simulink model "bhaaa"  (R2016b)
settings: Solver=ode15s  StartTime=0.0  StopTime=30  FixedStep=0.001  RelTol=1e-5  EnableMultiTasking=on
undefined symbols (not defined in the file): b1_damp, b2_damp, b3_damp, b4_damp, g, Hz, L1x, L1y, L1z, L2x, L2y, L2z, L3x, L3y, L3z, mass1, mass2, mass3, mass4, Rturn, sigbuilder_block, theta1_0, theta1_dot_0, theta2_0, theta2_dot_0, theta3_0, theta3_dot_0, theta4_0, theta4_dot_0, X, Y, Z
libraries: sm_lib x26, nesl_utility x17
(part 2 of 2)

== matlab function bhaaa/SIMULINK_MODEL/inside_MCKGQ/MCKGQ ==
  data: L1X_s input; M output; L2X_s input; L3X_s input; L1Y_s input; L2Y_s input; L3Y_s input; L1Z_s input; L2Z_s input; L3Z_s input; R4_s input; TH1_s input; TH2_s input; TH3_s input; TH1_s_D input; TH2_s_D input; TH3_s_D input; TH4_s_D input; b1_s input; b2_s input; b3_s input; b4_s input; g_s input; m1_s input; m2_s input; m3_s input; m4_s input; taum1_s input; taum2_s input; taum3_s input; taum4_s input; C output; K output; G output; Q output
function [M,C,K,G,Q] = MCKGQ(L1X_s,L2X_s,L3X_s,L1Y_s,L2Y_s,L3Y_s,L1Z_s,L2Z_s,L3Z_s,R4_s,TH1_s,TH2_s,TH3_s,TH1_s_D,TH2_s_D,TH3_s_D,TH4_s_D,b1_s,b2_s,b3_s,b4_s,g_s,m1_s,m2_s,m3_s,m4_s,taum1_s,taum2_s,taum3_s,taum4_s)
%#codegen

%    This function was generated by the Symbolic Math Toolbox version 7.0.
%    13-Sep-2016 13:01:16

M = reshape([L1Y_s.^2.*m1_s.*(1.0./3.0)+L1Y_s.^2.*m2_s+L1Y_s.^2.*m3_s+L2Y_s.^2.*m2_s.*(1.0./3.0)+L2Y_s.^2.*m3_s+L3Y_s.^2.*m3_s.*(1.0./3.0)+L1Z_s.^2.*m1_s.*(1.0./1.2e1)+L2Z_s.^2.*m2_s.*(1.0./1.2e1)+L3Z_s.^2.*m3_s.*(1.0./1.2e1)+L1Y_s.*L2Y_s.*m2_s.*cos(TH2_s)+L1Y_s.*L2Y_s.*m3_s.*cos(TH2_s).*2.0+L2Y_s.*L3Y_s.*m3_s.*cos(TH3_s)+L1Y_s.*L3Y_s.*m3_s.*cos(TH2_s+TH3_s),L2Y_s.^2.*m2_s.*(1.0./3.0)+L2Y_s.^2.*m3_s+L3Y_s.^2.*m3_s.*(1.0./3.0)+L2Z_s.^2.*m2_s.*(1.0./1.2e1)+L3Z_s.^2.*m3_s.*(1.0./1.2e1)+L1Y_s.*L2Y_s.*m2_s.*cos(TH2_s).*(1.0./2.0)+L1Y_s.*L2Y_s.*m3_s.*cos(TH2_s)+L2Y_s.*L3Y_s.*m3_s.*cos(TH3_s)+L1Y_s.*L3Y_s.*m3_s.*cos(TH2_s+TH3_s).*(1.0./2.0),m3_s.*(L3Y_s.^2.*4.0+L3Z_s.^2+L1Y_s.*L3Y_s.*cos(TH2_s+TH3_s).*6.0+L2Y_s.*L3Y_s.*cos(TH3_s).*6.0).*(1.0./1.2e1),0.0,L2Y_s.^2.*m2_s.*(1.0./3.0)+L2Y_s.^2.*m3_s+L3Y_s.^2.*m3_s.*(1.0./3.0)+L2Z_s.^2.*m2_s.*(1.0./1.2e1)+L3Z_s.^2.*m3_s.*(1.0./1.2e1)+L1Y_s.*L2Y_s.*m2_s.*cos(TH2_s).*(1.0./2.0)+L1Y_s.*L2Y_s.*m3_s.*cos(TH2_s)+L2Y_s.*L3Y_s.*m3_s.*cos(TH3_s)+L1Y_s.*L3Y_s.*m3_s.*cos(TH2_s+TH3_s).*(1.0./2.0),L2Y_s.^2.*m2_s.*(1.0./3.0)+L2Y_s.^2.*m3_s+L3Y_s.^2.*m3_s.*(1.0./3.0)+L2Z_s.^2.*m2_s.*(1.0./1.2e1)+L3Z_s.^2.*m3_s.*(1.0./1.2e1)+L2Y_s.*L3Y_s.*m3_s.*cos(TH3_s),m3_s.*(L3Y_s.^2.*4.0+L3Z_s.^2+L2Y_s.*L3Y_s.*cos(TH3_s).*6.0).*(1.0./1.2e1),0.0,m3_s.*(L3Y_s.^2.*4.0+L3Z_s.^2+L1Y_s.*L3Y_s.*cos(TH2_s+TH3_s).*6.0+L2Y_s.*L3Y_s.*cos(TH3_s).*6.0).*(1.0./1.2e1),m3_s.*(L3Y_s.^2.*4.0+L3Z_s.^2+L2Y_s.*L3Y_s.*cos(TH3_s).*6.0).*(1.0./1.2e1),m3_s.*(L3Y_s.^2.*4.0+L3Z_s.^2).*(1.0./1.2e1),0.0,0.0,0.0,0.0,L1X_s.^2.*m1_s.*(1.0./1.2e1)+L2X_s.^2.*m2_s.*(1.0./1.2e1)+L3X_s.^2.*m3_s.*(1.0./1.2e1)+L1Y_s.^2.*m1_s.*(1.0./6.0)+L1Y_s.^2.*m2_s.*(1.0./2.0)+L1Y_s.^2.*m3_s.*(1.0./2.0)+L2Y_s.^2.*m2_s.*(1.0./6.0)+L2Y_s.^2.*m3_s.*(1.0./2.0)+L3Y_s.^2.*m3_s.*(1.0./6.0)+L1Z_s.^2.*m1_s.*(1.0./2.4e1)+L2Z_s.^2.*m2_s.*(1.0./2.4e1)+L3Z_s.^2.*m3_s.*(1.0./2.4e1)+R4_s.^2.*m4_s.*(1.0./2.0)+L3Y_s.^2.*m3_s.*cos(TH1_s.*2.0+TH2_s.*2.0+TH3_s.*2.0).*(1.0./6.0)-L3Z_s.^2.*m3_s.*cos(TH1_s.*2.0+TH2_s.*2.0+TH3_s.*2.0).*(1.0./2.4e1)+L1Y_s.^2.*m1_s.*cos(TH1_s.*2.0).*(1.0./6.0)+L1Y_s.^2.*m2_s.*cos(TH1_s.*2.0).*(1.0./2.0)+L1Y_s.^2.*m3_s.*cos(TH1_s.*2.0).*(1.0./2.0)-L1Z_s.^2.*m1_s.*cos(TH1_s.*2.0).*(1.0./2.4e1)+L2Y_s.^2.*m2_s.*cos(TH1_s.*2.0+TH2_s.*2.0).*(1.0./6.0)+L2Y_s.^2.*m3_s.*cos(TH1_s.*2.0+TH2_s.*2.0).*(1.0./2.0)-L2Z_s.^2.*m2_s.*cos(TH1_s.*2.0+TH2_s.*2.0).*(1.0./2.4e1)+L1Y_s.*L2Y_s.*m2_s.*cos(TH2_s).*(1.0./2.0)+L1Y_s.*L2Y_s.*m3_s.*cos(TH2_s)+L2Y_s.*L3Y_s.*m3_s.*cos(TH3_s).*(1.0./2.0)+L1Y_s.*L2Y_s.*m2_s.*cos(TH1_s.*2.0+TH2_s).*(1.0./2.0)+L1Y_s.*L2Y_s.*m3_s.*cos(TH1_s.*2.0+TH2_s)+L1Y_s.*L3Y_s.*m3_s.*cos(TH1_s.*2.0+TH2_s+TH3_s).*(1.0./2.0)+L1Y_s.*L3Y_s.*m3_s.*cos(TH2_s+TH3_s).*(1.0./2.0)+L2Y_s.*L3Y_s.*m3_s.*cos(TH1_s.*2.0+TH2_s.*2.0+TH3_s).*(1.0./2.0)],[4,4]);
if nargout > 1
    C = reshape([-L1Y_s.*L3Y_s.*TH2_s_D.*m3_s.*sin(TH2_s+TH3_s)-L1Y_s.*L3Y_s.*TH3_s_D.*m3_s.*sin(TH2_s+TH3_s)-L1Y_s.*L2Y_s.*TH2_s_D.*m2_s.*sin(TH2_s)-L1Y_s.*L2Y_s.*TH2_s_D.*m3_s.*sin(TH2_s).*2.0-L2Y_s.*L3Y_s.*TH3_s_D.*m3_s.*sin(TH3_s),L1Y_s.*L3Y_s.*TH1_s_D.*m3_s.*sin(TH2_s+TH3_s).*(1.0./2.0)+L1Y_s.*L2Y_s.*TH1_s_D.*m2_s.*sin(TH2_s).*(1.0./2.0)+L1Y_s.*L2Y_s.*TH1_s_D.*m3_s.*sin(TH2_s)-L2Y_s.*L3Y_s.*TH3_s_D.*m3_s.*sin(TH3_s),L3Y_s.*m3_s.*(L1Y_s.*TH1_s_D.*sin(TH2_s+TH3_s)+L2Y_s.*TH1_s_D.*sin(TH3_s)+L2Y_s.*TH2_s_D.*sin(TH3_s).*2.0).*(1.0./2.0),TH4_s_D.*(L3Y_s.^2.*m3_s.*sin(TH1_s.*2.0+TH2_s.*2.0+TH3_s.*2.0).*4.0-L3Z_s.^2.*m3_s.*sin(TH1_s.*2.0+TH2_s.*2.0+TH3_s.*2.0)+L1Y_s.^2.*m1_s.*sin(TH1_s.*2.0).*4.0+L1Y_s.^2.*m2_s.*sin(TH1_s.*2.0).*1.2e1+L1Y_s.^2.*m3_s.*sin(TH1_s.*2.0).*1.2e1-L1Z_s.^2.*m1_s.*sin(TH1_s.*2.0)+L2Y_s.^2.*m2_s.*sin(TH1_s.*2.0+TH2_s.*2.0).*4.0+L2Y_s.^2.*m3_s.*sin(TH1_s.*2.0+TH2_s.*2.0).*1.2e1-L2Z_s.^2.*m2_s.*sin(TH1_s.*2.0+TH2_s.*2.0)+L1Y_s.*L2Y_s.*m2_s.*sin(TH1_s.*2.0+TH2_s).*1.2e1+L1Y_s.*L2Y_s.*m3_s.*sin(TH1_s.*2.0+TH2_s).*2.4e1+L1Y_s.*L3Y_s.*m3_s.*sin(TH1_s.*2.0+TH2_s+TH3_s).*1.2e1+L2Y_s.*L3Y_s.*m3_s.*sin(TH1_s.*2.0+TH2_s.*2.0+TH3_s).*1.2e1).*(-1.0./1.2e1),L1Y_s.*L3Y_s.*TH2_s_D.*m3_s.*sin(TH2_s+TH3_s).*(-1.0./2.0)-L1Y_s.*L3Y_s.*TH3_s_D.*m3_s.*sin(TH2_s+TH3_s)-L1Y_s.*L2Y_s.*TH2_s_D.*m2_s.*sin(TH2_s).*(1.0./2.0)-L1Y_s.*L2Y_s.*TH2_s_D.*m3_s.*sin(TH2_s)-L2Y_s.*L3Y_s.*TH3_s_D.*m3_s.*sin(TH3_s),-L2Y_s.*L3Y_s.*TH3_s_D.*m3_s.*sin(TH3_s),L2Y_s.*L3Y_s.*TH2_s_D.*m3_s.*sin(TH3_s).*(1.0./2.0),TH4_s_D.*(L3Y_s.^2.*m3_s.*sin(TH1_s.*2.0+TH2_s.*2.0+TH3_s.*2.0).*4.0-L3Z_s.^2.*m3_s.*sin(TH1_s.*2.0+TH2_s.*2.0+TH3_s.*2.0)+L2Y_s.^2.*m2_s.*sin(TH1_s.*2.0+TH2_s.*2.0).*4.0+L2Y_s.^2.*m3_s.*sin(TH1_s.*2.0+TH2_s.*2.0).*1.2e1-L2Z_s.^2.*m2_s.*sin(TH1_s.*2.0+TH2_s.*2.0)+L1Y_s.*L2Y_s.*m2_s.*sin(TH2_s).*6.0+L1Y_s.*L2Y_s.*m3_s.*sin(TH2_s).*1.2e1+L1Y_s.*L2Y_s.*m2_s.*sin(TH1_s.*2.0+TH2_s).*6.0+L1Y_s.*L2Y_s.*m3_s.*sin(TH1_s.*2.0+TH2_s).*1.2e1+L1Y_s.*L3Y_s.*m3_s.*sin(TH1_s.*2.0+TH2_s+TH3_s).*6.0+L1Y_s.*L3Y_s.*m3_s.*sin(TH2_s+TH3_s).*6.0+L2Y_s.*L3Y_s.*m3_s.*sin(TH1_s.*2.0+TH2_s.*2.0+TH3_s).*1.2e1).*(-1.0./1.2e1),L3Y_s.*TH3_s_D.*m3_s.*(L1Y_s.*sin(TH2_s+TH3_s)+L2Y_s.*sin(TH3_s)).*(-1.0./2.0),L2Y_s.*L3Y_s.*TH3_s_D.*m3_s.*sin(TH3_s).*(-1.0./2.0),0.0,TH4_s_D.*m3_s.*(L3Y_s.^2.*sin(TH1_s.*2.0+TH2_s.*2.0+TH3_s.*2.0).*4.0-L3Z_s.^2.*sin(TH1_s.*2.0+TH2_s.*2.0+TH3_s.*2.0)+L1Y_s.*L3Y_s.*sin(TH1_s.*2.0+TH2_s+TH3_s).*6.0+L1Y_s.*L3Y_s.*sin(TH2_s+TH3_s).*6.0+L2Y_s.*L3Y_s.*sin(TH1_s.*2.0+TH2_s.*2.0+TH3_s).*6.0+L2Y_s.*L3Y_s.*sin(TH3_s).*6.0).*(-1.0./1.2e1),TH4_s_D.*(L3Y_s.^2.*m3_s.*sin(TH1_s.*2.0+TH2_s.*2.0+TH3_s.*2.0).*4.0-L3Z_s.^2.*m3_s.*sin(TH1_s.*2.0+TH2_s.*2.0+TH3_s.*2.0)+L1Y_s.^2.*m1_s.*sin(TH1_s.*2.0).*4.0+L1Y_s.^2.*m2_s.*sin(TH1_s.*2.0).*1.2e1+L1Y_s.^2.*m3_s.*sin(TH1_s.*2.0).*1.2e1-L1Z_s.^2.*m1_s.*sin(TH1_s.*2.0)+L2Y_s.^2.*m2_s.*sin(TH1_s.*2.0+TH2_s.*2.0).*4.0+L2Y_s.^2.*m3_s.*sin(TH1_s.*2.0+TH2_s.*2.0).*1.2e1-L2Z_s.^2.*m2_s.*sin(TH1_s.*2.0+TH2_s.*2.0)+L1Y_s.*L2Y_s.*m2_s.*sin(TH1_s.*2.0+TH2_s).*1.2e1+L1Y_s.*L2Y_s.*m3_s.*sin(TH1_s.*2.0+TH2_s).*2.4e1+L1Y_s.*L3Y_s.*m3_s.*sin(TH1_s.*2.0+TH2_s+TH3_s).*1.2e1+L2Y_s.*L3Y_s.*m3_s.*sin(TH1_s.*2.0+TH2_s.*2.0+TH3_s).*1.2e1).*(1.0./2.4e1),TH4_s_D.*(L3Y_s.^2.*m3_s.*sin(TH1_s.*2.0+TH2_s.*2.0+TH3_s.*2.0).*4.0-L3Z_s.^2.*m3_s.*sin(TH1_s.*2.0+TH2_s.*2.0+TH3_s.*2.0)+L2Y_s.^2.*m2_s.*sin(TH1_s.*2.0+TH2_s.*2.0).*4.0+L2Y_s.^2.*m3_s.*sin(TH1_s.*2.0+TH2_s.*2.0).*1.2e1-L2Z_s.^2.*m2_s.*sin(TH1_s.*2.0+TH2_s.*2.0)+L1Y_s.*L2Y_s.*m2_s.*sin(TH2_s).*6.0+L1Y_s.*L2Y_s.*m3_s.*sin(TH2_s).*1.2e1+L1Y_s.*L2Y_s.*m2_s.*sin(TH1_s.*2.0+TH2_s).*6.0+L1Y_s.*L2Y_s.*m3_s.*sin(TH1_s.*2.0+TH2_s).*1.2e1+L1Y_s.*L3Y_s.*m3_s.*sin(TH1_s.*2.0+TH2_s+TH3_s).*6.0+L1Y_s.*L3Y_s.*m3_s.*sin(TH2_s+TH3_s).*6.0+L2Y_s.*L3Y_s.*m3_s.*sin(TH1_s.*2.0+TH2_s.*2.0+TH3_s).*1.2e1).*(1.0./2.4e1),TH4_s_D.*m3_s.*(L3Y_s.^2.*sin(TH1_s.*2.0+TH2_s.*2.0+TH3_s.*2.0).*4.0-L3Z_s.^2.*sin(TH1_s.*2.0+TH2_s.*2.0+TH3_s.*2.0)+L1Y_s.*L3Y_s.*sin(TH1_s.*2.0+TH2_s+TH3_s).*6.0+L1Y_s.*L3Y_s.*sin(TH2_s+TH3_s).*6.0+L2Y_s.*L3Y_s.*sin(TH1_s.*2.0+TH2_s.*2.0+TH3_s).*6.0+L2Y_s.*L3Y_s.*sin(TH3_s).*6.0).*(1.0./2.4e1),0.0],[4,4]);
end
if nargout > 2
    K = reshape([0.0,0.0,0.0,0.0,0.0,0.0,0.0,0.0,0.0,0.0,0.0,0.0,0.0,0.0,0.0,0.0],[4,4]);
end
if nargout > 3
    G = [g_s.*(L2Y_s.*m2_s.*cos(TH1_s+TH2_s)+L2Y_s.*m3_s.*cos(TH1_s+TH2_s).*2.0+L1Y_s.*m1_s.*cos(TH1_s)+L1Y_s.*m2_s.*cos(TH1_s).*2.0+L1Y_s.*m3_s.*cos(TH1_s).*2.0+L3Y_s.*m3_s.*cos(TH1_s+TH2_s+TH3_s)).*(1.0./2.0);L3Y_s.*g_s.*m3_s.*cos(TH1_s+TH2_s+TH3_s).*(1.0./2.0)+L2Y_s.*g_s.*m2_s.*cos(TH1_s+TH2_s).*(1.0./2.0)+L2Y_s.*g_s.*m3_s.*cos(TH1_s+TH2_s);L3Y_s.*g_s.*m3_s.*cos(TH1_s+TH2_s+TH3_s).*(1.0./2.0);0.0];
end
if nargout > 4
    Q = [taum1_s-TH1_s_D.*b1_s;taum2_s-TH2_s_D.*b2_s;taum3_s-TH3_s_D.*b3_s;taum4_s-TH4_s_D.*b4_s];
end

== matlab function bhaaa/SIMULINK_MODEL/inside_MCKGQ/Subsystem1/MATLAB Function ==
  data: M input; the_cond output
function the_cond = COND(M)
%#codegen

the_cond = cond(M);

end
